simulink model "det3x3_BB_HDL"  (R2024a)
settings: Solver=VariableStepAuto  StartTime=0.0  StopTime=200e-9  RelTol=1e-3
undefined symbols (not defined in the file or in its folder): S, vsva2197, xcvc1902
libraries: hdlBasic x4, hdlSSR x1, hdlUtilities x1, vmcUtilities x1
settings Model: Creator=catalinb  LastModifiedBy=sdegala
settings DebuggingCC: UnconnectedInputMsg=warning  UnconnectedOutputMsg=warning  UnconnectedLineMsg=warning
settings ModelReferenceCC: EnableRefExpFcnMdlSchedulingChecks=on
settings RTWCC: GPUComputeCapability=3.5  DLArmComputeVersion=19.05

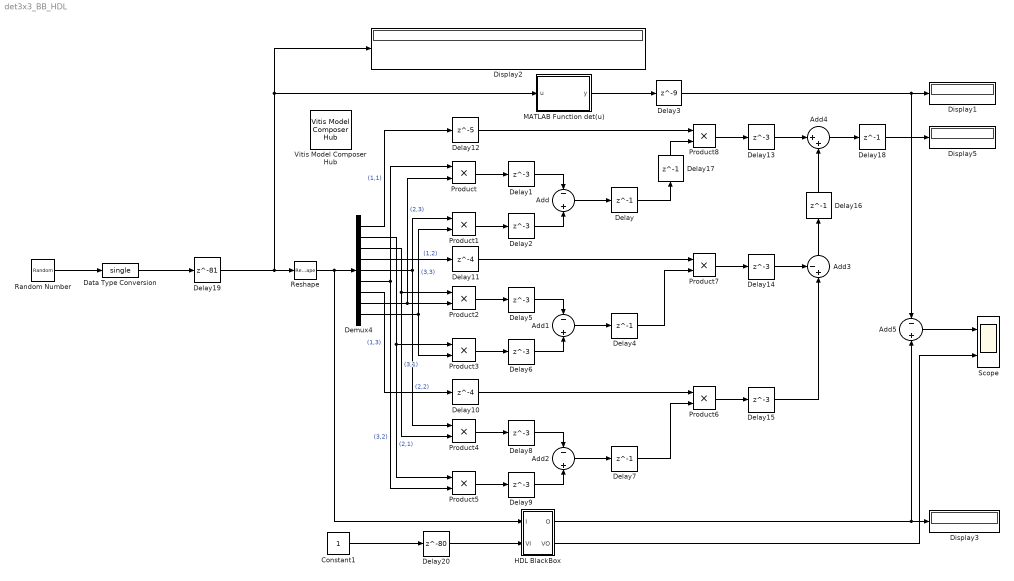
== system det3x3_BB_HDL ==
  Add{,1..2,5} (4 alike) : Sum  Inputs=-|+
  Add3 : Sum  Inputs=-+|
  Add4 : Sum  Inputs=|++
  Constant1 : Constant  OutDataTypeStr=single  SampleTime=1/805e6
  Data Type Conversion : DataTypeConversion  OutDataTypeStr=single  SaturateOnIntegerOverflow=off  RndMeth=Floor
  Delay{,4,7,16..18} (6 alike) : Delay  DelayLength=1
  Delay{1..2,5..6,8..9,13..15} (9 alike) : Delay  DelayLength=3
  Delay10 : Delay  DelayLength=4
  Delay11 : Delay  DelayLength=4
  Delay12 : Delay  DelayLength=5
  Delay19 : Delay  DelayLength=81
  Delay20 : Delay  DelayLength=80
  Delay3 : Delay  DelayLength=9
  Demux4 : Demux  Outputs=9
  Display{1..3,5} (4 alike) : Display
  HDL BlackBox : Subsystem
  MATLAB Function det(u) : MATLAB Function  TreatAsAtomicUnit=on
  Product{,1..8} (9 alike) : Product
  Random Number : RandomNumber  Mean=zeros(3,3)  Variance=ones(3,3)  Seed=reshape(1:9,3,3)  SampleTime=1.242e-9  VectorParams1D=off
  Reshape : Reshape
  Scope : Scope  NumInputPorts=2
  Vitis Model Composer Hub : vmcUtilities/Vitis Model Composer Hub  Tag=genX  CodeGeneration=off  SubsystemName=HDL BlackBox  BlockHierPath=det3x3_BB_HDL/HDL BlackBox  CompilationType=HDLCompilation  SubsystemType=HDLNode  ExportTypeV2=IP Catalog  StartColumn=1  NumberOfColumns=1  TargetDirectory=./netlist  exportDesign=on  analyzeDesign=off  validateDesignOnHw=off  ExportType=AI Engines  IpVendor=xilinx.com  IpLibrary=hls  IpVersion=1.0  IpHWLanguage=Verilog  AieCompilerOptions={}  AieSimulatorOptions={}  CreateTestbench=off  TestbenchStackSize=10  RunRtlSim=off  RunCSim=off  RunAieSim=off  AieSimTimeout=50000  RunAieSimProfiling=off  LaunchVitisAnalyzer=off  PlotOutput=off  RunX86Sim=off  X86SimTimeout=10  GenHwImage=off  GenLibadfXo=on  GenHwValidationCode=off  PlatformType=Specify Platform  Platform=/proj/xbuilds/SWIP/9999.0_0905_1841/installs/lin64/2025.2/Vitis/base_platforms/xilinx_vck190_base_202520_1/xilinx_vck190_base_202520_1.xpfm  HwSystemType=Baremetal  HwValidationTarget=hw  ProjDevice=Versal VCK190 Evaluation Platform (xcvc1902-vsva2197-2MP-e-S)  ProjDevicePart=xcvc1902-vsva2197-2MP-e-S  AIEType=AIE  SamplePeriod=-1  ClockFrequency=200  DataPathParallelism=1  xilinxfamily=versalaicore  part=xcvc1902  speed=-2MP-e-S  package=vsva2197  directory=./netlist/ip/HDLBlackBox/src  testbench=off  incr_netlist=off  synthesis_tool=Vivado  clock_wrapper=Clock Enables  dbl_ovrd=According to Block Masks  dcm_input_clock_period=10  sysclk_period=1.242  simulink_period=1.242e-9  eval_field=0  IPInfoJsonString="{\"DUTSubsystemName\":\"HDL\\nBlackBox\",\"HDLSubsystem\":{\"SubsystemName\":\"HDL_BlackBox\",\"IPName\":\"Subsystem\",\"IPLibrary\":\"VMC\",\"IPVendor\":\"User Company\",\"IPVersion\":\"1.0\",\"TargetDirectory\":\"./netlist\",\"SubsystemDir\":\"./netlist/ip/HDL_BlackBox\",\"FreqHz\":\"805152979.066\"},\"SubsystemTag\":\"HDLNode\"}"  LogFileName=/proj/xhdhdstaff5/sdegala/Head1/HEAD/ModelComposer_Sept16/Vitis_Model_Composer/Examples/HDL/Floating_Point/3x3_Matrix_Determinant/netlist/model_composer.log  NThreads=4  IPConfigFile=/tmp/vmctmp-9769773316677438567/det3x3_BB_HDL_ipconfig.json
  wires:
  Add/1 -> Delay/1
  Product/1 -> Delay1/1
  Delay1/1 -> Add/1
  Product1/1 -> Delay2/1
  Delay2/1 -> Add/2
  Delay/1 -> Delay17/1
  MATLAB Function det(u)/1(y) -> Delay3/1
  Delay3/1 -> Add5/1, Display1/1
  Reshape/1 -> HDL BlackBox/1(" I "), Demux4/1
  Demux4/1 -> Delay12/1  "(1,1)"
  Demux4/4 -> Delay11/1  "(1,2)"
  Demux4/7 -> Delay10/1  "(1,3)"
  Demux4/2 -> Product3/1, Product5/1  "(2,1)"
  Demux4/5 -> Product4/1, Product1/1  "(2,2)"
  Demux4/9 -> Product3/2, Product1/2  "(3,3)"
  Demux4/6 -> Product/1, Product5/2  "(3,2)"
  Demux4/8 -> Product/2, Product2/2  "(2,3)"
  Random Number/1 -> Data Type Conversion/1
  Delay4/1 -> Product7/2
  Delay6/1 -> Add1/2
  Product3/1 -> Delay6/1
  Delay5/1 -> Add1/1
  Product2/1 -> Delay5/1
  Add1/1 -> Delay4/1
  Demux4/3 -> Product4/2, Product2/1  "(3,1)"
  Add2/1 -> Delay7/1
  Product4/1 -> Delay8/1
  Delay8/1 -> Add2/1
  Product5/1 -> Delay9/1
  Delay9/1 -> Add2/2
  Delay7/1 -> Product6/2
  Delay10/1 -> Product6/1
  Delay11/1 -> Product7/1
  Delay12/1 -> Product8/1
  Product8/1 -> Delay13/1
  Product7/1 -> Delay14/1
  Product6/1 -> Delay15/1
  Delay14/1 -> Add3/1
  Delay15/1 -> Add3/2
  Add4/1 -> Delay18/1
  Delay16/1 -> Add4/2
  Add3/1 -> Delay16/1
  Delay13/1 -> Add4/1
  Delay18/1 -> Display5/1
  Delay17/1 -> Product8/2
  Delay20/1 -> HDL BlackBox/2(" VI ")
  HDL BlackBox/1(" O ") -> Add5/2, Display3/1
  Add5/1 -> Scope/1
  Delay19/1 -> MATLAB Function det(u)/1(u), Display2/1, Reshape/1
  Data Type Conversion/1 -> Delay19/1
  Constant1/1 -> Delay20/1
  HDL BlackBox/2(" VO ") -> Scope/2

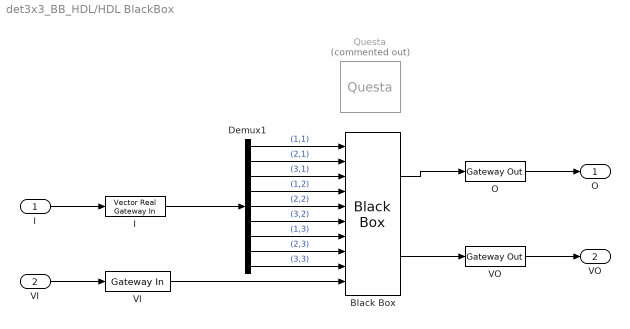
== system det3x3_BB_HDL/HDL BlackBox ==
  " I " : Inport
  " VI " : Inport  Port=2
  Black Box : hdlBasic/Black Box  init_code=DET3x3_config  sim_method=Vivado Simulator  verbose=off  XmcBlockStatus=1  maskContainerNames=group1  block_type=blackbox2  block_config=sysgen:black_box_config
  Demux1 : Demux  Outputs=9
  I : hdlSSR/Vector Real Gateway In  gui_display_data_type=Floating-point  arith_type=Floating-point  n_bits=16  bin_pt=14  preci_type=Single  exp_width=8  frac_width=24  quantization="Round  (unbiased: +/- Inf)"  overflow=Saturate  period=1.242e-9  sg_ssr=9  UseAsADC=off  ADCChannel='1'  interface=None  automatic_assignment=on  address_offset=hex2dec('00')  intf_name=''  intf_description=''  default_value=0  timing_constraint=None  locs_specified=off  LOCs={}  io_standard={}  inherit_from_input=off  hdl_port=on  interface_prev=1  block_type=realgatewayin_ssr  XmcBlockStatus=1  sg_ssr_prev=9  maskContainerNames=group4  block_width_w=590  block_height_w=670  block_width=640  block_height=850
  O : hdlBasic/Gateway Out  inherit_from_input=on  bool_to_boolean=off  hdl_port=on  rows=1  columns=1  UseAsDAC=off  DACChannel='1'  interface=None  automatic_assignment=on  address_offset=hex2dec('00')  intf_name=''  intf_description=''  timing_constraint=None  locs_specified=off  LOCs={}  io_standard={}  XmcBlockStatus=1  maskContainerNames=group4  block_type=gatewayout  block_config=sysgen:gateway_out_config  block_width_w=590  block_height_w=620  block_width=620  block_height=750
  Questa : hdlUtilities/Questa  Commented=on  startup_timeout=40  block_type=hdlcosim  XmcBlockStatus=0  maskContainerNames=Container4  dir=./questa  waveform=on  leave_open=on  skip_compile=off  map_unisim_lib=on  unisim_lib_path=C:\Xilinx\Vivado\2022.2\compile_simlib\questa  use_unisim=on  custom_scripts=on  post_vsim_script=wave.do
  VI : hdlBasic/Gateway In  gui_display_data_type=Boolean  arith_type=Boolean  n_bits=16  bin_pt=14  preci_type=Single  exp_width=8  frac_width=24  rows=1  columns=1  quantization="Round  (unbiased: +/- Inf)"  overflow=Saturate  period=1.242e-9  UseAsADC=off  ADCChannel='1'  interface=None  automatic_assignment=on  address_offset=hex2dec('00')  intf_name=''  intf_description=''  default_value=0  timing_constraint=None  locs_specified=off  LOCs={}  io_standard={}  inherit_from_input=off  hdl_port=on  XmcBlockStatus=1  maskContainerNames=group4  block_type=gatewayin  block_config=sysgen:gateway_in_config  block_width_w=590  block_height_w=620  block_width=640  block_height=850
  VO : hdlBasic/Gateway Out  inherit_from_input=off  bool_to_boolean=off  hdl_port=on  rows=1  columns=1  UseAsDAC=off  DACChannel='1'  interface=None  automatic_assignment=on  address_offset=hex2dec('00')  intf_name=''  intf_description=''  timing_constraint=None  locs_specified=off  LOCs={}  io_standard={}  XmcBlockStatus=1  maskContainerNames=group4  block_type=gatewayout  block_config=sysgen:gateway_out_config  block_width_w=590  block_height_w=620  block_width=620  block_height=750
  " O " : Outport
  " VO " : Outport  Port=2
  wires:
  Black Box/2 -> VO/1
  VI/1 -> Black Box/10
  Demux1/4 -> Black Box/4  "(1,2)"
  Demux1/5 -> Black Box/5  "(2,2)"
  Black Box/1 -> O/1
  Demux1/8 -> Black Box/8  "(2,3)"
  Demux1/7 -> Black Box/7  "(1,3)"
  Demux1/3 -> Black Box/3  "(3,1)"
  Demux1/1 -> Black Box/1  "(1,1)"
  I/1 -> Demux1/1
  Demux1/2 -> Black Box/2  "(2,1)"
  Demux1/9 -> Black Box/9  "(3,3)"
  Demux1/6 -> Black Box/6  "(3,2)"
  " I "/1 -> I/1
  " VI "/1 -> VI/1
  O/1 -> " O "/1
  VO/1 -> " VO "/1

== matlab function det3x3_BB_HDL/MATLAB Function det(u) ==
  data: u input; y output
function y = fcn(u)

y = det(u);
